simulink model "pitch"  (R2025b)
settings: Solver=FixedStepDiscrete  StartTime=0.0  StopTime=inf  RelTol=1e-3
undefined symbols (not defined in the file): Semitone_rt
settings Model: Creator=linogarciamorales  LastModifiedBy=linogarciamorales
settings OptimizationCC: EnhancedBackFolding=on  PassReuseOutputArgsAs=Individual arguments  ZeroExternalMemoryAtStartup=off  ZeroInternalMemoryAtStartup=off  OptimizeBlockOrder=speed  DifferentSizesBufferReuse=on  OptimizationCustomize=off  EfficientTunableParamExpr=on
settings DebuggingCC: ParameterTunabilityLossMsg=error
settings SFSimCC: MATLABDynamicMemAlloc=off
settings RTWCC: SystemTargetFile=ert.tlc  GenCodeOnly=on  TemplateMakefile=ert_default_tmf  Description=Embedded Coder
settings CodeAppCC: ForceParamTrailComments=on  IgnoreCustomStorageClasses=off  OperatorAnnotations=on  SimulinkDataObjDesc=on  SFDataObjDesc=on  InsertBlockDesc=on
settings ERTTargetCC: InlinedParameterPlacement=Hierarchical  ERTCustomFileTemplate=example_file_process.tlc  TargetLangStandard=C99 (ISO)  GenerateSampleERTMain=on  SupportNonInlinedSFcns=on

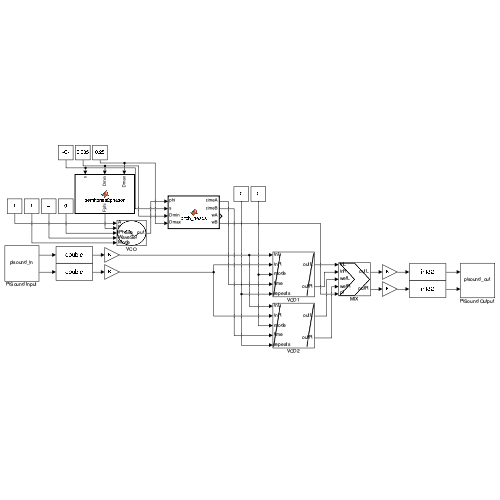
[thumbnail: Simulink's stored preview of the top-level diagram]
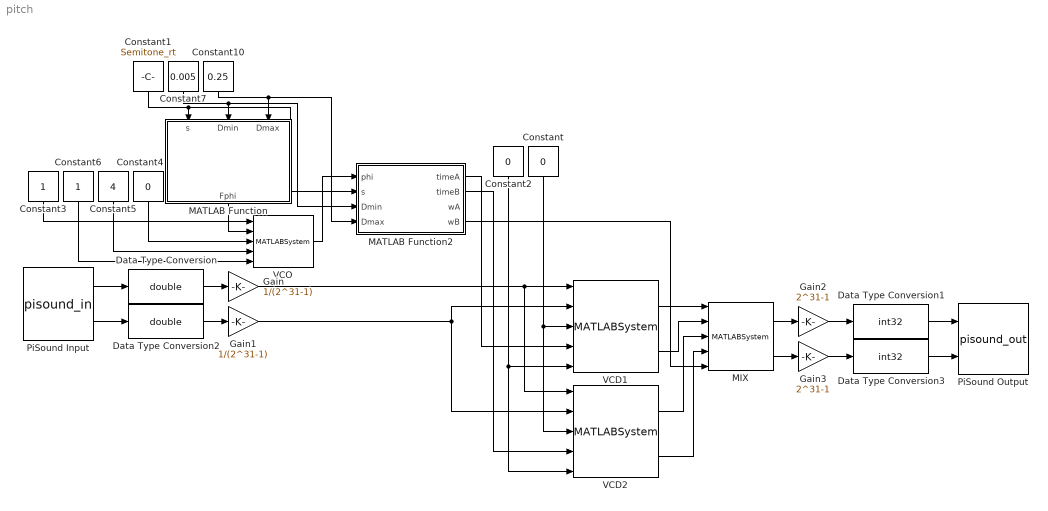
== system pitch ==
  Constant : Constant  Value=0  OutDataTypeStr=uint8
  Constant1 : Constant  Value=Semitone_rt  OutDataTypeStr=double
  Constant10 : Constant  Value=0.25  OutDataTypeStr=double
  Constant2 : Constant  Value=0  OutDataTypeStr=double
  Constant3 : Constant  OutDataTypeStr=double
  Constant4 : Constant  Value=0  OutDataTypeStr=double
  Constant5 : Constant  Value=4  OutDataTypeStr=uint8
  Constant6 : Constant  OutDataTypeStr=uint8
  Constant7 : Constant  Value=0.005  OutDataTypeStr=double
  Data Type Conversion : DataTypeConversion  OutDataTypeStr=double  SaturateOnIntegerOverflow=off  RndMeth=Floor
  Data Type Conversion1 : DataTypeConversion  OutDataTypeStr=int32  SaturateOnIntegerOverflow=off  RndMeth=Floor
  Data Type Conversion2 : DataTypeConversion  OutDataTypeStr=double  SaturateOnIntegerOverflow=off  RndMeth=Floor
  Data Type Conversion3 : DataTypeConversion  OutDataTypeStr=int32  SaturateOnIntegerOverflow=off  RndMeth=Floor
  Gain : Gain  Gain=1/(2^31-1)
  Gain1 : Gain  Gain=1/(2^31-1)
  Gain2 : Gain  Gain=2^31-1
  Gain3 : Gain  Gain=2^31-1
  MATLAB Function : MATLAB Function  TreatAsAtomicUnit=on
  MATLAB Function2 : MATLAB Function  TreatAsAtomicUnit=on
  MIX : MATLABSystem  System=mix_sys  N=128  Fs=48000  Mode=uint8(3)  SmoothTime=0.01  IndepInDB=false  SimulateUsing=Code generation
      mask Type: mix_sys
  PiSound Input : S-Function  FunctionName=pisound_in  Parameters=48000, 128, 0  SFunctionDeploymentMode=off  EnableBusSupport=off
  PiSound Output : S-Function  FunctionName=pisound_out  Parameters=48000, 128, 0  SFunctionDeploymentMode=off  EnableBusSupport=off
  VCD1 : MATLABSystem  System=vcd_sys  N=128  Fs=48000  MaxDelay=2  Mode=uint8(1)  Delay=0.1  g=0.5  SimulateUsing=Code generation
      mask Type: vcd_sys
  VCD2 : MATLABSystem  System=vcd_sys  N=128  Fs=48000  MaxDelay=2  Mode=uint8(1)  Delay=0.1  g=0.5  SimulateUsing=Code generation
      mask Type: vcd_sys
  VCO : MATLABSystem  System=vco_mono_sys  N=128  Fs=48000  OutMaxL=4096  InFixL=1024  SimulateUsing=Code generation
      mask Type: vco_mono_sys
  wires:
  PiSound Input/1 -> Data Type Conversion/1
  PiSound Input/2 -> Data Type Conversion2/1
  Data Type Conversion1/1 -> PiSound Output/1
  Data Type Conversion3/1 -> PiSound Output/2
  Gain2/1 -> Data Type Conversion1/1
  Gain3/1 -> Data Type Conversion3/1
  Data Type Conversion/1 -> Gain/1
  Data Type Conversion2/1 -> Gain1/1
  Constant/1 -> VCD1/3, VCD2/3
  MATLAB Function/1(Fphi) -> VCO/2
  Constant3/1 -> VCO/1
  Constant4/1 -> VCO/3
  Constant5/1 -> VCO/4
  Constant6/1 -> VCO/5
  Constant2/1 -> VCD2/5, VCD1/5
  Constant1/1 -> MATLAB Function2/2(s), MATLAB Function/1(s)
  Constant10/1 -> MATLAB Function2/4(Dmax), MATLAB Function/3(Dmax)
  Constant7/1 -> MATLAB Function2/3(Dmin), MATLAB Function/2(Dmin)
  VCO/1 -> MATLAB Function2/1(phi)
  MATLAB Function2/1(timeA) -> VCD1/4
  MATLAB Function2/2(timeB) -> VCD2/4
  Gain/1 -> VCD2/1, VCD1/1
  Gain1/1 -> VCD2/2, VCD1/2
  MATLAB Function2/4(wB) -> MIX/5
  MIX/2 -> Gain3/1
  VCD1/1 -> MIX/1
  VCD1/2 -> MIX/2
  VCD2/1 -> MIX/3
  VCD2/2 -> MIX/4
  MIX/1 -> Gain2/1

== matlab function pitch/MATLAB Function ==
  data: s input; Fphi output; Dmin input; Dmax input
function Fphi = semitones2phasor(s, Dmin, Dmax)
% s en semitonos, Dmin/Dmax en segundos
Dspan = Dmax - Dmin;
if Dspan <= 0
  Fphi = 0; 
  return;
end

r = 2^(s/12);

if abs(r-1) < 1e-6
  Fphi = 0;   % (o muy pequeño) y puedes fijar wA=1, wB=0
else
  Fphi = abs(r-1)/Dspan;
end
end

== matlab function pitch/MATLAB Function2 ==
  data: phi input; timeA output; s input; Dmin input; Dmax input; timeB output; wA output; wB output
function [timeA,timeB,wA,wB] = pitch_heads(phi, s, Dmin, Dmax)
    % phi: [N x 1] en [0,1)
    % s: semitonos (scalar)
    % Dmin/Dmax: segundos (scalar)
    Dspan = Dmax - Dmin;
    % segundo head: phiB = mod(phi+0.5,1)
    phiB = phi + 0.5;
    phiB = phiB - floor(phiB);
    % ventanas (crossfade)
    wA = 0.5*(1 - cos(2*pi*phi));
    wB = 1 - wA;
    % mapping fase -> retardo (segundos)
    if s >= 0
        timeA = Dmax - phi .* Dspan; timeB = Dmax - phiB .* Dspan;
        % pitch up
    else
        timeA = Dmin + phi .* Dspan; timeB = Dmin + phiB .* Dspan;
        % pitch down
    end
end
